simulink model "sla_iir_filter"  (R2015b)
settings: Solver=FixedStepDiscrete  SolverMode=SingleTasking  StartTime=0.0  StopTime=10.0  RelTol=1e-3
PreLoadFcn:
  | edit design_iir_filter
undefined symbols (not defined in the file or in its folder): dfilt
libraries: simulink x1, dsparch4 x1
settings Model: Creator=at-mt  LastModifiedBy=amatsumo
settings DataIOCC: SaveFormat=Array  SignalLoggingSaveFormat=ModelDataLogs  SaveOutput=off  SignalLogging=off  SaveTime=off
settings OptimizationCC: BlockReduction=off  ConditionallyExecuteInputs=off  DefaultParameterBehavior=Inlined  ExpressionDepthLimit=2147483647
settings DebuggingCC: AlgebraicLoopMsg=error  UnderspecifiedInitializationDetection=Classic  MergeDetectMultiDrivingBlocksExec=none  SolverPrmCheckMsg=warning  SingleTaskRateTransMsg=error  ParameterOverflowMsg=warning  FcnCallInpInsideContextMsg=UseLocalSettings  StateNameClashWarn=warning
settings HardwareCC: ProdBitPerPointer=32  ProdLargestAtomicFloat=None  ProdIntDivRoundTo=Undefined  ProdEndianess=Unspecified  ProdWordSize=32  ProdHWDeviceType=ASIC/FPGA->ASIC/FPGA  ProdEqTarget=off
settings GRTTargetCC: GeneratePreprocessorConditionals=Disable all  CombineOutputUpdateFcns=off  GRTInterface=on
settings ConfigComp: CovModelRefEnable=Off  CovSFcnEnable=off

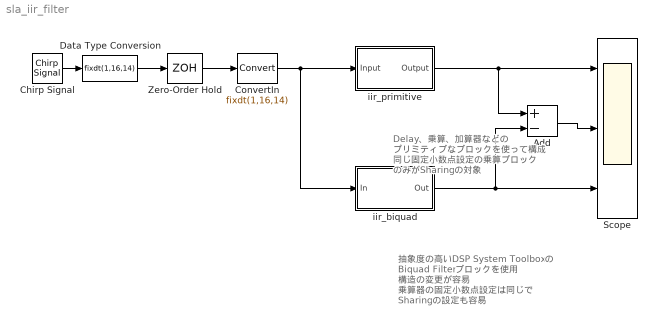
== system sla_iir_filter ==
  note: 抽象度の高いDSP System Toolboxの
      | Biquad Filterブロックを使用
      | 構造の変更が容易
      | 乗算器の固定小数点設定は同じで
      | Sharingの設定も容易
  note: Delay、乗算、加算器などの
      | プリミティブなブロックを使って構成
      | 同じ固定小数点設定の乗算ブロック
      | のみがSharingの対象
  Add : Sum  Inputs=+-
  Chirp Signal : simulink/Sources/Chirp Signal  f1=10  T=10  f2=500
  ConvertIn : DataTypeConversion  OutDataTypeStr=fixdt(1,16,14)  RndMeth=Nearest  SaturateOnIntegerOverflow=on
  Data Type Conversion : DataTypeConversion  OutDataTypeStr=fixdt(1,16,14)  RndMeth=Nearest
  Scope : Scope  NumInputPorts=3
  Zero-Order Hold : ZeroOrderHold  SampleTime=1/1000
  iir_biquad : Subsystem  Tag=BlockMethodSubSystem
  iir_primitive : Subsystem  Tag=FilterWizardSubSystem
      settings: ErrorFcn=dspFilterRealizedInBasicElemsAlgLoopErrFcnCallback
  wires:
  Chirp Signal/1 -> Data Type Conversion/1
  Zero-Order Hold/1 -> ConvertIn/1
  iir_biquad/1(Out) -> Scope/3, Add/2
  Add/1 -> Scope/2
  Data Type Conversion/1 -> Zero-Order Hold/1
  iir_primitive/1(Output) -> Add/1, Scope/1
  ConvertIn/1 -> iir_biquad/1(In), iir_primitive/1(Input)

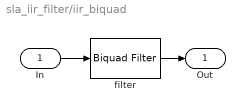
== system sla_iir_filter/iir_biquad ==
  In : Inport
  filter : dsparch4/Biquad Filter  IIRFiltStruct=Direct form I  CoeffSource=Specify via dialog  BiQuadCoeffs=[0.24409398394376244 0.24638056656065699 0 1 -0.50952544949558054 0;0.062065195388954407 0.12485735055712442 0.062797610475028798 1 -1.0578315579506707 0.30755171437177825;0.070025174293722847 0.13975985825982012 0.069740858362236438 1 -1.1840906753873925 0.46361656630317183;0.085165513395946066 0.16888899552149816 0.083731006821812726 1 -1.430882406486973 0.76866792222623082]  a0Flag=Warning  IC=0  ICnum=0  ICden=0  InputProcessing=Columns as channels (frame based)  firstCoeffMode=Binary point scaling  firstCoeffWordLength=18  firstCoeffFracLength=19  outputMode=Binary point scaling  outputWordLength=16  outputFracLength=14  accumMode=Binary point scaling  accumWordLength=40  accumFracLength=33  denAccumFracLength=30  prodOutputMode=Binary point scaling  prodOutputWordLength=34  prodOutputFracLength=33  denProdOutputFracLength=30  secondMemoryFracLength=15  roundingMode=Convergent  overflowMode=off  ScaleValues=[1;1;1;1;1.0000000000006222]  optimizeScaleValues=on  ScaleValueMode=Specify via input port (g)  scaleValueFracLength=17  stageInputMode=Binary point scaling  stageOutputMode=Binary point scaling  stageInputWordLength=16  stageInputFracLength=14  stageOutputWordLength=16  stageOutputFracLength=14  FilterSource=Specify via dialog  FilterObject=dfilt.df2tsos([1 0.3 0.4],[1 0.1 0.2])
  Out : Outport
  wires:
  In/1 -> filter/1
  filter/1 -> Out/1

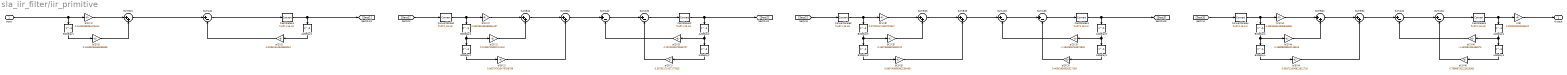
== system sla_iir_filter/iir_primitive ==
  Input : Inport
  A2Delay{1..4} (4 alike) : Delay  DelayLength=1  InitialCondition=0
  A3Delay2 : Delay  DelayLength=1  InitialCondition=0
  A3Delay3 : Delay  DelayLength=1  InitialCondition=0
  A3Delay4 : Delay  DelayLength=1  InitialCondition=0
  B2Delay{1..4} (4 alike) : Delay  DelayLength=1  InitialCondition=0
  B3Delay2 : Delay  DelayLength=1  InitialCondition=0
  B3Delay3 : Delay  DelayLength=1  InitialCondition=0
  B3Delay4 : Delay  DelayLength=1  InitialCondition=0
  CastStates{1..4} (4 alike) : DataTypeConversion  OutDataTypeStr=fixdt(1,16,14)  RndMeth=Convergent
  ConvertScale2 : DataTypeConversion  OutDataTypeStr=fixdt(1,16,14)  RndMeth=Convergent
  ConvertScale3 : DataTypeConversion  OutDataTypeStr=fixdt(1,16,14)  RndMeth=Convergent
  ConvertScale4 : DataTypeConversion  OutDataTypeStr=fixdt(1,16,14)  RndMeth=Convergent
  SumA{21..24,32..34} (7 alike) : Sum  Inputs=|+-  AccumDataTypeStr=fixdt(1,40,30)  OutDataTypeStr=fixdt(1,40,30)  RndMeth=Convergent
  SumB{21..24,32..34} (7 alike) : Sum  Inputs=|++  AccumDataTypeStr=fixdt(1,40,33)  OutDataTypeStr=fixdt(1,40,33)  RndMeth=Convergent
  a(2)(1) : Gain  Gain=-0.50952544949558054  ParamDataTypeStr=fixdt(1,18,16)  OutDataTypeStr=fixdt(1,34,30)  RndMeth=Convergent
  a(2)(2) : Gain  Gain=-1.0578315579506707  ParamDataTypeStr=fixdt(1,18,16)  OutDataTypeStr=fixdt(1,34,30)  RndMeth=Convergent
  a(2)(3) : Gain  Gain=-1.1840906753873925  ParamDataTypeStr=fixdt(1,18,16)  OutDataTypeStr=fixdt(1,34,30)  RndMeth=Convergent
  a(2)(4) : Gain  Gain=-1.430882406486973  ParamDataTypeStr=fixdt(1,18,16)  OutDataTypeStr=fixdt(1,34,30)  RndMeth=Convergent
  a(3)(2) : Gain  Gain=0.30755171437177825  ParamDataTypeStr=fixdt(1,18,16)  OutDataTypeStr=fixdt(1,34,30)  RndMeth=Convergent
  a(3)(3) : Gain  Gain=0.46361656630317183  ParamDataTypeStr=fixdt(1,18,16)  OutDataTypeStr=fixdt(1,34,30)  RndMeth=Convergent
  a(3)(4) : Gain  Gain=0.76866792222623082  ParamDataTypeStr=fixdt(1,18,16)  OutDataTypeStr=fixdt(1,34,30)  RndMeth=Convergent
  b(1)(1) : Gain  Gain=0.24409398394376244  ParamDataTypeStr=fixdt(1,18,19)  OutDataTypeStr=fixdt(1,34,33)  RndMeth=Convergent
  b(1)(2) : Gain  Gain=0.062065195388954407  ParamDataTypeStr=fixdt(1,18,19)  OutDataTypeStr=fixdt(1,34,33)  RndMeth=Convergent
  b(1)(3) : Gain  Gain=0.070025174293722847  ParamDataTypeStr=fixdt(1,18,19)  OutDataTypeStr=fixdt(1,34,33)  RndMeth=Convergent
  b(1)(4) : Gain  Gain=0.085165513395946066  ParamDataTypeStr=fixdt(1,18,19)  OutDataTypeStr=fixdt(1,34,33)  RndMeth=Convergent
  b(2)(1) : Gain  Gain=0.24638056656065699  ParamDataTypeStr=fixdt(1,18,19)  OutDataTypeStr=fixdt(1,34,33)  RndMeth=Convergent
  b(2)(2) : Gain  Gain=0.12485735055712442  ParamDataTypeStr=fixdt(1,18,19)  OutDataTypeStr=fixdt(1,34,33)  RndMeth=Convergent
  b(2)(3) : Gain  Gain=0.13975985825982012  ParamDataTypeStr=fixdt(1,18,19)  OutDataTypeStr=fixdt(1,34,33)  RndMeth=Convergent
  b(2)(4) : Gain  Gain=0.16888899552149816  ParamDataTypeStr=fixdt(1,18,19)  OutDataTypeStr=fixdt(1,34,33)  RndMeth=Convergent
  b(3)(2) : Gain  Gain=0.062797610475028798  ParamDataTypeStr=fixdt(1,18,19)  OutDataTypeStr=fixdt(1,34,33)  RndMeth=Convergent
  b(3)(3) : Gain  Gain=0.069740858362236438  ParamDataTypeStr=fixdt(1,18,19)  OutDataTypeStr=fixdt(1,34,33)  RndMeth=Convergent
  b(3)(4) : Gain  Gain=0.083731006821812726  ParamDataTypeStr=fixdt(1,18,19)  OutDataTypeStr=fixdt(1,34,33)  RndMeth=Convergent
  s(5) : Gain  Gain=1.0000000000006222  ParamDataTypeStr=fixdt(1,18,17)  OutDataTypeStr=fixdt(1,16,14)  RndMeth=Convergent
  Output : Outport
  wires:
  Input/1 -> b(1)(1)/1, B2Delay1/1
  b(1)(1)/1 -> SumB21/1
  SumB21/1 -> SumA21/1
  SumA21/1 -> CastStates1/1
  CastStates1/1 -> [Sect1], A2Delay1/1
  B2Delay1/1 -> b(2)(1)/1
  b(2)(1)/1 -> SumB21/2
  a(2)(1)/1 -> SumA21/2
  A2Delay1/1 -> a(2)(1)/1
  [Sect1] -> ConvertScale2/1
  ConvertScale2/1 -> b(1)(2)/1, B2Delay2/1
  b(1)(2)/1 -> SumB22/1
  SumB22/1 -> SumB32/1
  SumB32/1 -> SumA22/1
  SumA22/1 -> SumA32/1
  SumA32/1 -> CastStates2/1
  CastStates2/1 -> [Sect2], A2Delay2/1
  B2Delay2/1 -> b(2)(2)/1, B3Delay2/1
  b(2)(2)/1 -> SumB22/2
  a(2)(2)/1 -> SumA22/2
  A2Delay2/1 -> a(2)(2)/1, A3Delay2/1
  B3Delay2/1 -> b(3)(2)/1
  b(3)(2)/1 -> SumB32/2
  a(3)(2)/1 -> SumA32/2
  A3Delay2/1 -> a(3)(2)/1
  [Sect2] -> ConvertScale3/1
  ConvertScale3/1 -> b(1)(3)/1, B2Delay3/1
  b(1)(3)/1 -> SumB23/1
  SumB23/1 -> SumB33/1
  SumB33/1 -> SumA23/1
  SumA23/1 -> SumA33/1
  SumA33/1 -> CastStates3/1
  CastStates3/1 -> [Sect3], A2Delay3/1
  B2Delay3/1 -> b(2)(3)/1, B3Delay3/1
  b(2)(3)/1 -> SumB23/2
  a(2)(3)/1 -> SumA23/2
  A2Delay3/1 -> a(2)(3)/1, A3Delay3/1
  B3Delay3/1 -> b(3)(3)/1
  b(3)(3)/1 -> SumB33/2
  a(3)(3)/1 -> SumA33/2
  A3Delay3/1 -> a(3)(3)/1
  [Sect3] -> ConvertScale4/1
  ConvertScale4/1 -> b(1)(4)/1, B2Delay4/1
  b(1)(4)/1 -> SumB24/1
  SumB24/1 -> SumB34/1
  SumB34/1 -> SumA24/1
  SumA24/1 -> SumA34/1
  SumA34/1 -> CastStates4/1
  CastStates4/1 -> s(5)/1, A2Delay4/1
  B2Delay4/1 -> b(2)(4)/1, B3Delay4/1
  b(2)(4)/1 -> SumB24/2
  a(2)(4)/1 -> SumA24/2
  A2Delay4/1 -> a(2)(4)/1, A3Delay4/1
  B3Delay4/1 -> b(3)(4)/1
  b(3)(4)/1 -> SumB34/2
  a(3)(4)/1 -> SumA34/2
  A3Delay4/1 -> a(3)(4)/1
  s(5)/1 -> Output/1
